simulink model "ACT_MAG"  (Simulink 9.0)
settings: Solver=VariableStepAuto  StartTime=0.0  StopTime=10.0  RelTol=1e-3
undefined symbols (not defined in the file or in its folder): ACT_MAG
settings Model: SuppressorTable=22 serialization::archive 11 0 6 0 0 0 0 0  Creator=Mahal  LastModifiedBy=WilTravis
settings DataIOCC: SaveFormat=Dataset
settings OptimizationCC: LifeSpan=auto
settings DebuggingCC: UnderspecifiedInitializationDetection=Simplified  MergeDetectMultiDrivingBlocksExec=error  SFUnexpectedBacktrackingDiag=error  SFNoUnconditionalDefaultTransitionDiag=error  SFExecutionAtInitializationDiag=warning
settings HardwareCC: ProdBitPerPointer=64  ProdBitPerSizeT=64  ProdBitPerPtrDiffT=64  ProdLargestAtomicFloat=Float  ProdIntDivRoundTo=Zero  ProdEndianess=LittleEndian  ProdWordSize=64  ProdHWDeviceType=Intel->x86-64 (Windows64)
settings ModelReferenceCC: PropagateSignalLabelsOutOfModel=on
settings CodeAppCC: StateflowObjectComments=off
settings GRTTargetCC: TargetLangStandard=C99 (ISO)
settings ConfigComp: CovMetricSettings=dwe  CovHtmlReporting=off  CovSaveCumulativeToWorkspaceVar=off  CovSaveSingleToWorkspaceVar=off  CovExternalEMLEnable=on

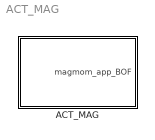
== system ACT_MAG ==
  ACT_MAG : Subsystem

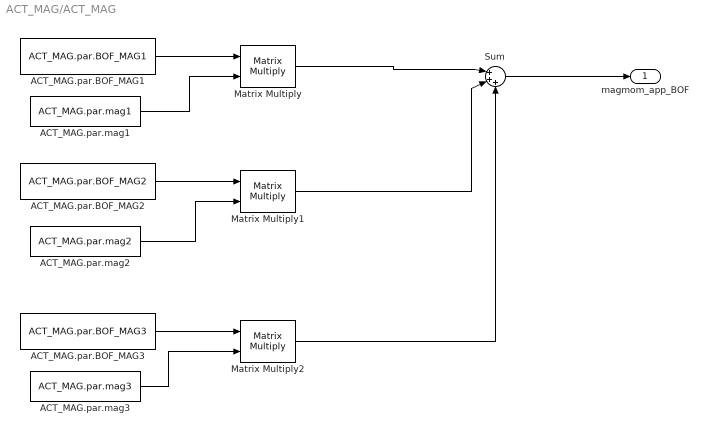
== system ACT_MAG/ACT_MAG ==
  ACT_MAG.par.BOF_MAG1 : Constant  Value=ACT_MAG.par.BOF_MAG1
  ACT_MAG.par.BOF_MAG2 : Constant  Value=ACT_MAG.par.BOF_MAG2
  ACT_MAG.par.BOF_MAG3 : Constant  Value=ACT_MAG.par.BOF_MAG3
  ACT_MAG.par.mag1 : Constant  Value=ACT_MAG.par.mag1
  "ACT_MAG.par.mag2 " : Constant  Value=ACT_MAG.par.mag2
  ACT_MAG.par.mag3 : Constant  Value=ACT_MAG.par.mag3
  Matrix Multiply : Product  Multiplication=Matrix(*)
  Matrix Multiply1 : Product  Multiplication=Matrix(*)
  Matrix Multiply2 : Product  Multiplication=Matrix(*)
  Sum : Sum  Inputs=|+++
  magmom_app_BOF : Outport
  wires:
  Sum/1 -> magmom_app_BOF/1
  ACT_MAG.par.mag1/1 -> Matrix Multiply/2
  "ACT_MAG.par.mag2 "/1 -> Matrix Multiply1/2
  Matrix Multiply/1 -> Sum/1
  ACT_MAG.par.mag3/1 -> Matrix Multiply2/2
  Matrix Multiply2/1 -> Sum/3
  Matrix Multiply1/1 -> Sum/2
  ACT_MAG.par.BOF_MAG3/1 -> Matrix Multiply2/1
  ACT_MAG.par.BOF_MAG1/1 -> Matrix Multiply/1
  ACT_MAG.par.BOF_MAG2/1 -> Matrix Multiply1/1
